simulink model "H4_34"  (R2021b)
settings: Solver=VariableStepAuto  StartTime=0.0  StopTime=10.0  RelTol=1e-3
libraries: dspsrcs4 x1
settings Model: Creator=DELL  LastModifiedBy=DELL

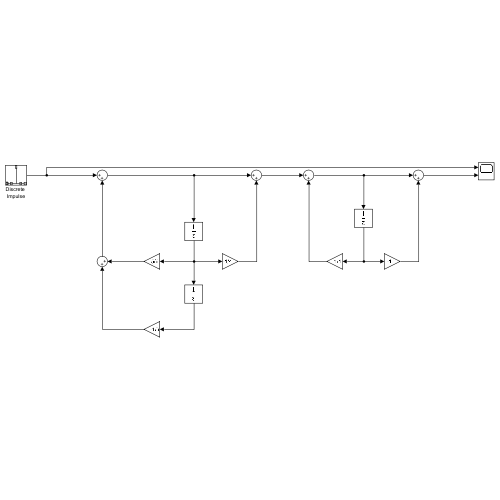
[thumbnail: Simulink's stored preview of the top-level diagram]
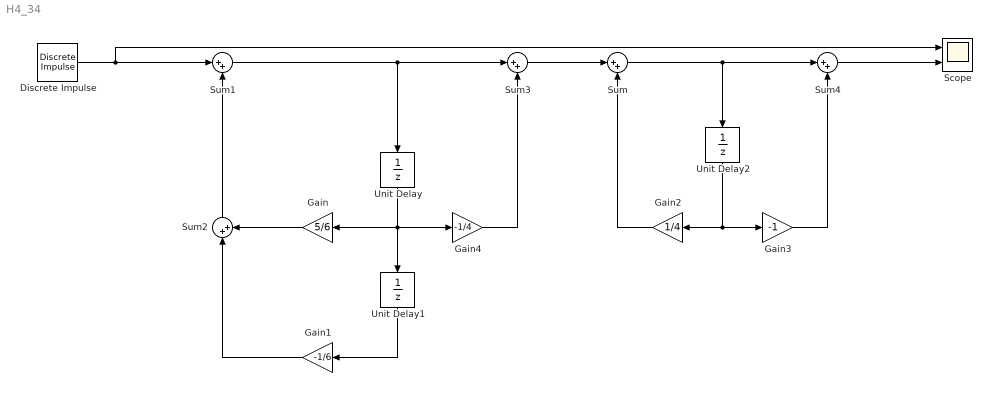
== system H4_34 ==
  Discrete Impulse : dspsrcs4/Discrete  Impulse  Delay=0  SampleTime=1  FrameSample=1  OutputFrames=off  dataType=double  isSigned=on  wordLen=16  udDataType=sfix(16)  fracBitsMode=Best precision  numFracBits=15  OutDataTypeStr=double  LastOutDataTypeStr=double
  Gain : Gain  Gain=5/6
  Gain1 : Gain  Gain=-1/6
  Gain2 : Gain  Gain=1/4
  Gain3 : Gain  Gain=-1
  Gain4 : Gain  Gain=-1/4
  Scope : Scope  NumInputPorts=2
  Sum{,1..4} (5 alike) : Sum  Inputs=|++
  Unit Delay : UnitDelay  SampleTime=-1  HasFrameUpgradeWarning=on
  Unit Delay1 : UnitDelay  SampleTime=-1  HasFrameUpgradeWarning=on
  Unit Delay2 : UnitDelay  SampleTime=-1  HasFrameUpgradeWarning=on
  wires:
  Gain/1 -> Sum2/2
  Sum2/1 -> Sum1/2
  Gain1/1 -> Sum2/1
  Unit Delay/1 -> Unit Delay1/1, Gain4/1, Gain/1
  Unit Delay1/1 -> Gain1/1
  Sum1/1 -> Unit Delay/1, Sum3/1
  Sum3/1 -> Sum/1
  Gain4/1 -> Sum3/2
  Gain2/1 -> Sum/2
  Sum/1 -> Sum4/1, Unit Delay2/1
  Unit Delay2/1 -> Gain3/1, Gain2/1
  Gain3/1 -> Sum4/2
  Discrete Impulse/1 -> Scope/1, Sum1/1
  Sum4/1 -> Scope/2
